simulink model "Forbilhastighed"  (Simulink 7.0)
settings: Solver=ode45  StartTime=0.0  StopTime=3000  RelTol=1e-5
libraries: simulink x2
settings Model: Creator=tom  LastModifiedBy=tom

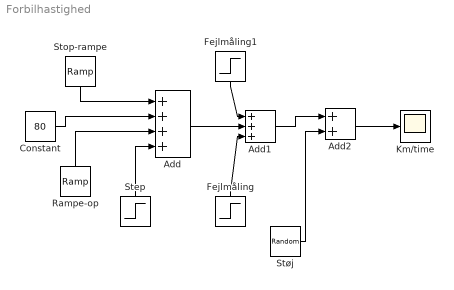
== system Forbilhastighed ==
  Add : Sum  Inputs=++++  OutDataType=sfix(16)  OutScaling=2^-10
  Add1 : Sum  Inputs=+++  OutDataType=sfix(16)  OutScaling=2^-10
  Add2 : Sum  OutDataType=sfix(16)  OutScaling=2^-10
  Constant : Constant  Value=80  OutDataType=sfix(16)  OutScaling=2^0
  Fejlmåling : Step  Orientation=up  Time=2000  After=-8  SampleTime=0
  Fejlmåling1 : Step  Orientation=down  Time=2010  After=8  SampleTime=0
  Km/time : Scope
  Rampe-op : simulink/Sources/Ramp  Orientation=up  SystemSampleTime=-1  slope=10/200  start=300  X0=0
  Step : Step  Orientation=up  Time=1000  After=-10  SampleTime=0
  Stop-rampe : simulink/Sources/Ramp  Orientation=down  SystemSampleTime=-1  slope=-10/200  start=500  X0=0
  Støj : RandomNumber  Variance=0.05  SampleTime=0
  wires:
  Step/1 -> Add/4
  Rampe-op/1 -> Add/3
  Constant/1 -> Add/2
  Stop-rampe/1 -> Add/1
  Fejlmåling/1 -> Add1/3
  Add/1 -> Add1/2
  Fejlmåling1/1 -> Add1/1
  Add1/1 -> Add2/1
  Add2/1 -> Km/time/1
  Støj/1 -> Add2/2
